simulink model "controller_2022"  (R2022b)
settings: Solver=ode4  StartTime=0.0  StopTime=500  FixedStep=0.001  RelTol=1e-3
model workspace (MAT data in the model file):
  x_0 = 0
values from neighbouring files (symbols this model uses):
  mode = 1    [run_sim.m]
  theta_ref = [0; pi/4; pi]    [run_sim.m]
  v_ref = [0;1;1]    [run_sim.m]
  x0 = zeros(21,1)    [eqn_motion.m]    (also in run_sim.m = zeros(22,1))
undefined symbols (not defined in the file or in its folder): para
libraries: simulink x11, cstblocks x3
settings Model: Creator=kiana  LastModifiedBy=kia241
settings DataIOCC: SaveOutput=off  SignalLogging=off  DSMLogging=off  SaveTime=off  ReturnWorkspaceOutputs=off  StateSaveName=xout_sim  TimeSaveName=tout_sim

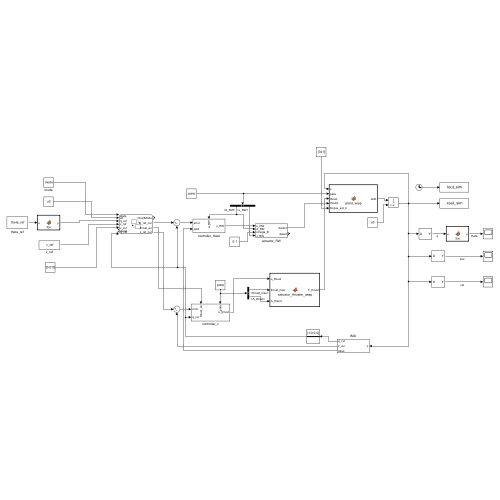
[thumbnail: Simulink's stored preview of the top-level diagram]
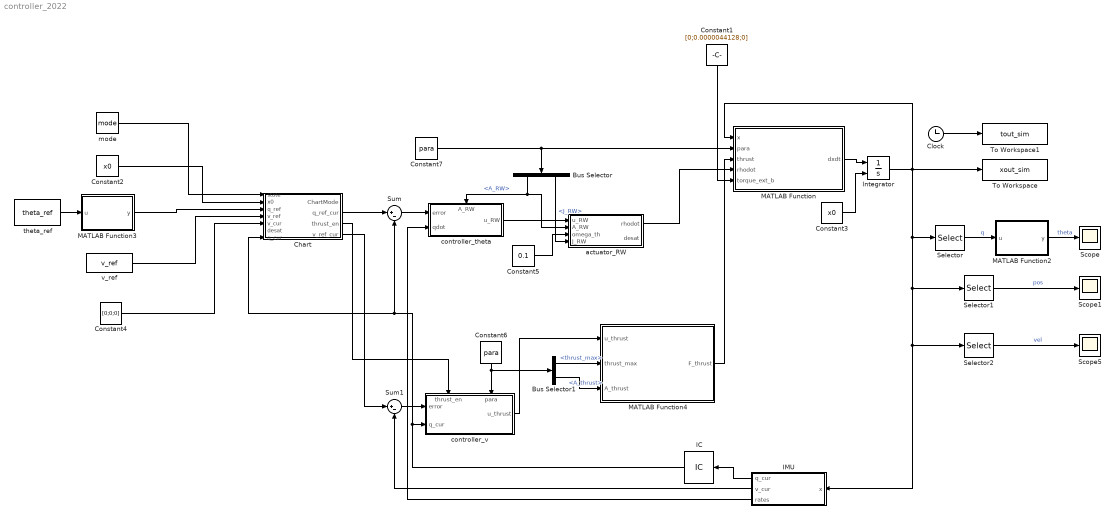
== system controller_2022 ==
  Bus Selector : BusSelector  OutputSignals=A_RW,J_RW
  Bus Selector1 : BusSelector  OutputSignals=thrust_max,A_thrust
  Chart : Stateflow chart  TreatAsAtomicUnit=on
      settings: PortSchema="{\"entries\":[{\"content\":{\"sides\":[{\"content\":{\"connectorIds\":[\"In1\",\"In2\",\"In4\",\"In5\",\"In6\",\"In7\",\"In3\"]},\"type\":\"ConnectorPlacement.EquallySpacedRectSide\",\"uuid\":\"521ec3b6-fc93-445b-ad1f-3cedbe1f933a\"},{\"content\":{\"connectorIds\":[\"Out1\",\"Out2\",\"Out3\",\"Out4\"],\"side\":\"RIGHT\"},\"type\":\"ConnectorPlacement.EquallySpacedRectSide\",\"uuid\":\"d47ee242-db22-486c-9cd8-a97188eab184\"},{\"content\":{\"side\":\"TOP\"},\"type\":\"ConnectorPlacement.EquallySpacedRectSide\",\"uuid\":\"3ac8246c-771a-4a3a-9153-436ad07c67be\"}]},\"type\":\"ConnectorPlacement.EquallySpacedConnector\",\"uuid\":\"e3bfbb62-b6a2-4288-b7fb-0587f308f30e\"}],\"packageUris\":[\"http://schema.mathworks.com/mf0/Connector/R2020b\"],\"version\":\"1.0\"}"
  Clock : Clock
  Constant1 : Constant  Value=[0;0.0000044128;0]
  Constant2 : Constant  Value=x0
  Constant3 : Constant  Value=x0
  Constant4 : Constant  Value=[0;0;0]
  Constant5 : Constant  Value=0.1
  Constant6 : Constant  Value=para  OutDataTypeStr=Bus: para_bus
  Constant7 : Constant  Value=para  OutDataTypeStr=Bus: para_bus
  IC : InitialCondition  Value=[1;0;0;0]
  IMU : Subsystem
  Integrator : Integrator  InitialConditionSource=external  InitialCondition=zeros(21,1)
  MATLAB Function : MATLAB Function  TreatAsAtomicUnit=on
  MATLAB Function2 : MATLAB Function  TreatAsAtomicUnit=on
  MATLAB Function3 : MATLAB Function  TreatAsAtomicUnit=on
  MATLAB Function4 : MATLAB Function  TreatAsAtomicUnit=on
  Scope : Scope
  Scope1 : Scope
  Scope5 : Scope
  Selector : Selector  InputPortWidth=22  IndexOptions=Index vector (dialog)  Indices=[1:4]  OutputSizes=1
  Selector1 : Selector  InputPortWidth=22  IndexOptions=Index vector (dialog)  Indices=[17:19]  OutputSizes=1
  Selector2 : Selector  InputPortWidth=22  IndexOptions=Index vector (dialog)  Indices=[20:22]  OutputSizes=1
  Sum : Sum  Inputs=|+-
  Sum1 : Sum  Inputs=|+-
  To Workspace : ToWorkspace  VariableName=xout_sim  SampleTime=-1
  To Workspace1 : ToWorkspace  VariableName=tout_sim  SampleTime=-1
  actuator_RW : Subsystem
  controller_theta : Subsystem
      settings: PortSchema="{\"entries\":[{\"content\":{\"sides\":[{\"content\":{\"connectorIds\":[\"In1\",\"In2\"]},\"type\":\"ConnectorPlacement.EquallySpacedRectSide\",\"uuid\":\"7526e81d-1261-4d66-9121-bc7373b2004f\"},{\"content\":{\"connectorIds\":[\"Out1\"],\"side\":\"RIGHT\"},\"type\":\"ConnectorPlacement.EquallySpacedRectSide\",\"uuid\":\"2fc2379f-a896-405a-8657-318c2691f466\"},{\"content\":{\"connectorIds\":[\"In3\"],\"side\":\"TOP\"},\"type\":\"ConnectorPlacement.EquallySpacedRectSide\",\"uuid\":\"3ebc5bb4-0a7b-439d-8491-5514c80b6d4e\"}]},\"type\":\"ConnectorPlacement.EquallySpacedConnector\",\"uuid\":\"e4bfc279-4423-461e-be0b-04258d5d0e38\"}],\"packageUris\":[\"http://schema.mathworks.com/mf0/Connector/R2020b\"],\"version\":\"1.0\"}"
  controller_v : Subsystem
      settings: PortSchema="{\"entries\":[{\"content\":{\"sides\":[{\"content\":{\"connectorIds\":[\"In1\",\"In2\"]},\"type\":\"ConnectorPlacement.EquallySpacedRectSide\",\"uuid\":\"7526e81d-1261-4d66-9121-bc7373b2004f\"},{\"content\":{\"connectorIds\":[\"Out1\"],\"side\":\"RIGHT\"},\"type\":\"ConnectorPlacement.EquallySpacedRectSide\",\"uuid\":\"2fc2379f-a896-405a-8657-318c2691f466\"},{\"content\":{\"connectorIds\":[\"In3\",\"In4\"],\"side\":\"TOP\"},\"type\":\"ConnectorPlacement.EquallySpacedRectSide\",\"uuid\":\"3ebc5bb4-0a7b-439d-8491-5514c80b6d4e\"}]},\"type\":\"ConnectorPlacement.EquallySpacedConnector\",\"uuid\":\"e4bfc279-4423-461e-be0b-04258d5d0e38\"}],\"packageUris\":[\"http://schema.mathworks.com/mf0/Connector/R2020b\"],\"version\":\"1.0\"}"
  mode : Constant  Value=mode
  theta_ref : Constant  Value=theta_ref
  v_ref : Constant  Value=v_ref
  wires:
  MATLAB Function/1(dxdt) -> Integrator/1
  MATLAB Function2/1(y) -> Scope/1  "theta"
  Constant3/1 -> Integrator/2
  Selector1/1 -> Scope1/1  "pos"
  Integrator/1 -> Selector2/1, IMU/1(x), Selector1/1, Selector/1, MATLAB Function/1(x), To Workspace/1
  IC/1 -> Chart/3(q_cur), Sum/2, controller_v/2(q_cur)
  Sum/1 -> controller_theta/1(error)
  controller_theta/1(u_RW) -> actuator_RW/1(u_RW)
  IMU/3(rates) -> controller_theta/2(qdot)
  v_ref/1 -> Chart/5(v_ref)
  IMU/2(v_cur) -> Sum1/2
  actuator_RW/1(rhodot) -> MATLAB Function/4(rhodot)
  Sum1/1 -> controller_v/1(error)
  Chart/4(v_ref_cur) -> Sum1/1
  mode/1 -> Chart/1(state)
  Constant2/1 -> Chart/2(x0)
  Selector/1 -> MATLAB Function2/1(u)  "q"
  Chart/2(q_ref_cur) -> Sum/1
  theta_ref/1 -> MATLAB Function3/1(u)
  MATLAB Function3/1(y) -> Chart/4(q_ref)
  IMU/1(q_cur) -> IC/1
  Constant1/1 -> MATLAB Function/5(torque_ext_b)
  Clock/1 -> To Workspace1/1
  MATLAB Function4/1(F_thrust) -> MATLAB Function/3(thrust)
  Selector2/1 -> Scope5/1  "vel"
  controller_v/1(u_thrust) -> MATLAB Function4/1(u_thrust)
  Chart/3(thrust_en) -> controller_v/3(thrust_en)
  Constant4/1 -> Chart/6(v_cur)
  Constant5/1 -> actuator_RW/3(omega_th)
  Constant7/1 -> MATLAB Function/2(para), Bus Selector/1
  Constant6/1 -> Bus Selector1/1, controller_v/4(para)
  Bus Selector/1 -> actuator_RW/2(A_RW), controller_theta/3(A_RW)  "<A_RW>"
  Bus Selector1/1 -> MATLAB Function4/2(thrust_max)  "<thrust_max>"
  Bus Selector1/2 -> MATLAB Function4/3(A_thrust)  "<A_thrust>"
  Bus Selector/2 -> actuator_RW/4(J_RW)  "<J_RW>"

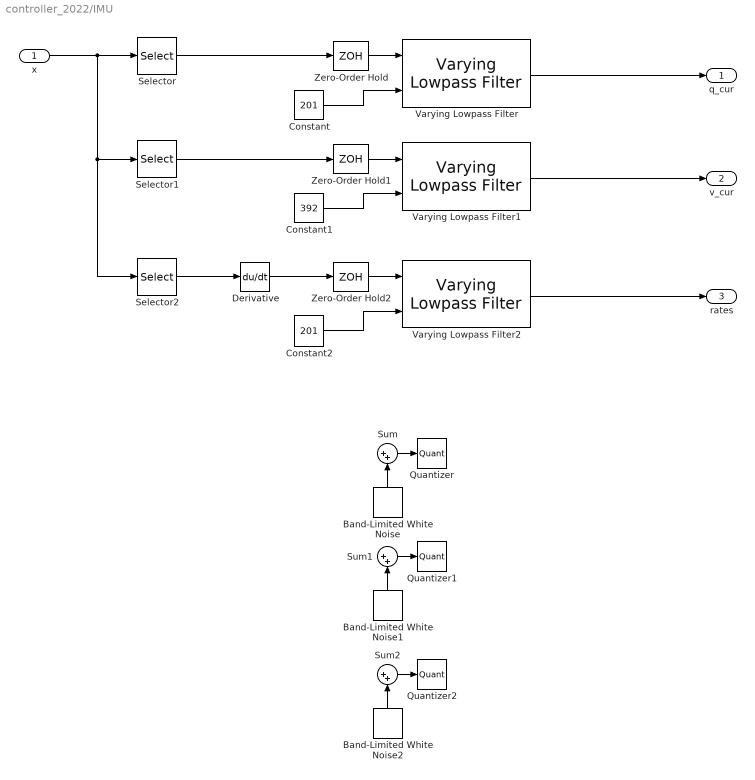
== system controller_2022/IMU ==
  x : Inport
  Band-Limited White Noise : simulink/Sources/Band-Limited White Noise  Cov=[0.1]  Ts=0.1  seed=[23341]
  Band-Limited White Noise1 : simulink/Sources/Band-Limited White Noise  Cov=[0.1]  Ts=0.1  seed=[23341]
  Band-Limited White Noise2 : simulink/Sources/Band-Limited White Noise  Cov=[0.1]  Ts=0.1  seed=[23341]
  Constant : Constant  Value=201
  Constant1 : Constant  Value=392
  Constant2 : Constant  Value=201
  Derivative : Derivative
  Quantizer : Quantizer
  Quantizer1 : Quantizer
  Quantizer2 : Quantizer
  Selector : Selector  InputPortWidth=22  IndexOptions=Index vector (dialog)  Indices=[1:4]  OutputSizes=1
  Selector1 : Selector  InputPortWidth=22  IndexOptions=Index vector (dialog)  Indices=[20:22]  OutputSizes=1
  Selector2 : Selector  InputPortWidth=22  IndexOptions=Index vector (dialog)  Indices=[1:4]  OutputSizes=1
  Sum : Sum  Inputs=|++
  Sum1 : Sum  Inputs=|++
  Sum2 : Sum  Inputs=|++
  Varying Lowpass Filter : cstblocks/Linear Parameter Varying/Varying Lowpass Filter  N=1
  Varying Lowpass Filter1 : cstblocks/Linear Parameter Varying/Varying Lowpass Filter  N=1
  Varying Lowpass Filter2 : cstblocks/Linear Parameter Varying/Varying Lowpass Filter  N=1
  Zero-Order Hold : ZeroOrderHold  SampleTime=0.01
  Zero-Order Hold1 : ZeroOrderHold  SampleTime=0.01
  Zero-Order Hold2 : ZeroOrderHold  SampleTime=0.01
  q_cur : Outport
  v_cur : Outport  Port=2
  rates : Outport  Port=3
  wires:
  x/1 -> Selector2/1, Selector1/1, Selector/1
  Selector/1 -> Zero-Order Hold/1
  Zero-Order Hold/1 -> Varying Lowpass Filter/1
  Constant/1 -> Varying Lowpass Filter/2
  Selector1/1 -> Zero-Order Hold1/1
  Zero-Order Hold1/1 -> Varying Lowpass Filter1/1
  Constant1/1 -> Varying Lowpass Filter1/2
  Constant2/1 -> Varying Lowpass Filter2/2
  Zero-Order Hold2/1 -> Varying Lowpass Filter2/1
  Selector2/1 -> Derivative/1
  Derivative/1 -> Zero-Order Hold2/1
  Sum/1 -> Quantizer/1
  Band-Limited White Noise/1 -> Sum/2
  Sum1/1 -> Quantizer1/1
  Band-Limited White Noise1/1 -> Sum1/2
  Sum2/1 -> Quantizer2/1
  Band-Limited White Noise2/1 -> Sum2/2
  Varying Lowpass Filter/1 -> q_cur/1
  Varying Lowpass Filter1/1 -> v_cur/1
  Varying Lowpass Filter2/1 -> rates/1

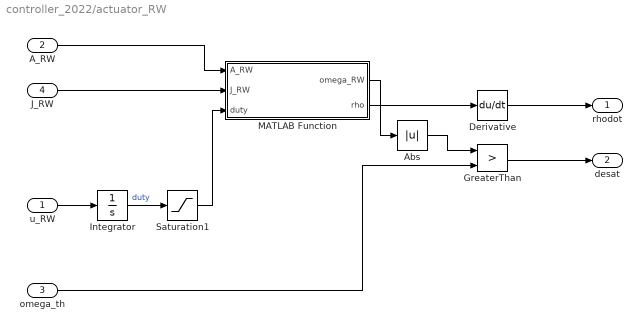
== system controller_2022/actuator_RW ==
  u_RW : Inport
  A_RW : Inport  Port=2
  omega_th : Inport  Port=3
  J_RW : Inport  Port=4
  Abs : Abs  SaturateOnIntegerOverflow=off
  Derivative : Derivative
  GreaterThan : RelationalOperator  Operator=>  OutDataTypeStr=boolean  RndMeth=Simplest  InputSameDT=off
  Integrator : Integrator  InitialCondition=0.15
  MATLAB Function : MATLAB Function  TreatAsAtomicUnit=on
  Saturation1 : Saturate  UpperLimit=0.2  LowerLimit=0.1
  rhodot : Outport
  desat : Outport  Port=2
  wires:
  omega_th/1 -> GreaterThan/2
  GreaterThan/1 -> desat/1
  A_RW/1 -> MATLAB Function/1(A_RW)
  MATLAB Function/2(rho) -> Derivative/1
  Derivative/1 -> rhodot/1
  J_RW/1 -> MATLAB Function/2(J_RW)
  MATLAB Function/1(omega_RW) -> Abs/1
  Abs/1 -> GreaterThan/1
  Integrator/1 -> Saturation1/1  "duty"
  Saturation1/1 -> MATLAB Function/3(duty)
  u_RW/1 -> Integrator/1

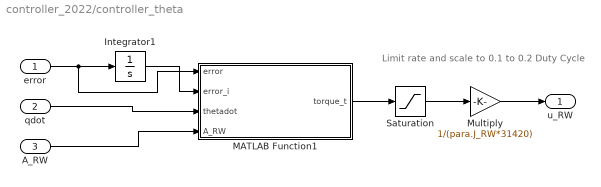
== system controller_2022/controller_theta ==
  note: Limit rate and scale to 0.1 to 0.2 Duty Cycle
  error : Inport
  qdot : Inport  Port=2
  A_RW : Inport  Port=3
  Integrator1 : Integrator  InitialCondition=[0;0;0;0]
  MATLAB Function1 : MATLAB Function  TreatAsAtomicUnit=on
  Multiply : Gain  Gain=1/(para.J_RW*31420)
  Saturation : Saturate  UpperLimit=0.018  LowerLimit=-0.018
  u_RW : Outport
  wires:
  error/1 -> Integrator1/1, MATLAB Function1/1(error)
  Integrator1/1 -> MATLAB Function1/2(error_i)
  A_RW/1 -> MATLAB Function1/4(A_RW)
  qdot/1 -> MATLAB Function1/3(thetadot)
  MATLAB Function1/1(torque_t) -> Saturation/1
  Multiply/1 -> u_RW/1
  Saturation/1 -> Multiply/1

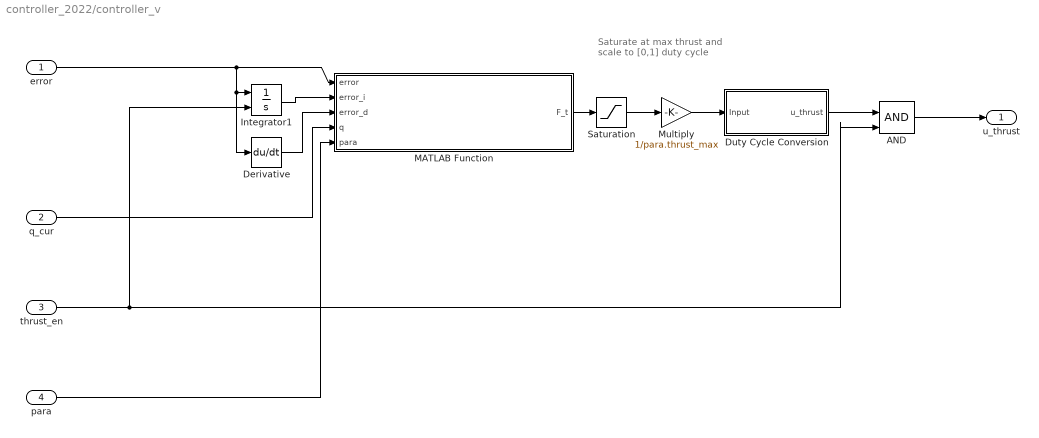
== system controller_2022/controller_v ==
  note: Saturate at max thrust and scale to [0,1] duty cycle
  error : Inport
  q_cur : Inport  Port=2
  thrust_en : Inport  Port=3
  para : Inport  Port=4
  AND : Logic  IconShape=distinctive  AllPortsSameDT=off  OutDataTypeStr=boolean
  Derivative : Derivative
  Duty Cycle Conversion : Subsystem
  Integrator1 : Integrator  ExternalReset=rising  InitialCondition=[0;0;0]
  MATLAB Function : MATLAB Function  TreatAsAtomicUnit=on
  Multiply : Gain  Gain=1/para.thrust_max
  Saturation : Saturate  UpperLimit=para.thrust_max  LowerLimit=0
  u_thrust : Outport
  wires:
  error/1 -> Derivative/1, Integrator1/1, MATLAB Function/1(error)
  Integrator1/1 -> MATLAB Function/2(error_i)
  Derivative/1 -> MATLAB Function/3(error_d)
  q_cur/1 -> MATLAB Function/4(q)
  MATLAB Function/1(F_t) -> Saturation/1
  AND/1 -> u_thrust/1
  Duty Cycle Conversion/1(u_thrust) -> AND/1
  thrust_en/1 -> Integrator1/2, AND/2
  Saturation/1 -> Multiply/1
  Multiply/1 -> Duty Cycle Conversion/1(Input)
  para/1 -> MATLAB Function/5(para)

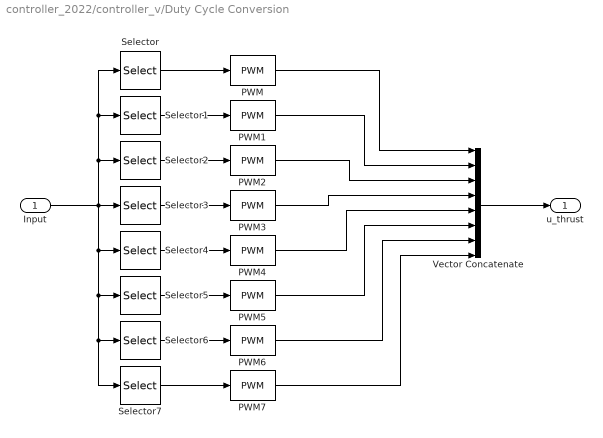
== system controller_2022/controller_v/Duty Cycle Conversion ==
  Input : Inport
  PWM : simulink/Discontinuities/PWM  DisableCoverage=on  Period=0.2  InitialDelay=0  DisallowZeroDutyCycle=off  RunAtFixedTimeIntervals=on  SampleTime=0.001
  PWM{1..7} (7 alike) : simulink/Discontinuities/PWM  DisableCoverage=on  Period=0.2  InitialDelay=0  DisallowZeroDutyCycle=off  RunAtFixedTimeIntervals=on  SampleTime=0.002
  Selector : Selector  InputPortWidth=8  IndexOptions=Index vector (dialog)  Indices=1  OutputSizes=1
  Selector1 : Selector  InputPortWidth=8  IndexOptions=Index vector (dialog)  Indices=2  OutputSizes=1
  Selector2 : Selector  InputPortWidth=8  IndexOptions=Index vector (dialog)  Indices=3  OutputSizes=1
  Selector3 : Selector  InputPortWidth=8  IndexOptions=Index vector (dialog)  Indices=4  OutputSizes=1
  Selector4 : Selector  InputPortWidth=8  IndexOptions=Index vector (dialog)  Indices=5  OutputSizes=1
  Selector5 : Selector  InputPortWidth=8  IndexOptions=Index vector (dialog)  Indices=6  OutputSizes=1
  Selector6 : Selector  InputPortWidth=8  IndexOptions=Index vector (dialog)  Indices=7  OutputSizes=1
  Selector7 : Selector  InputPortWidth=8  IndexOptions=Index vector (dialog)  Indices=8  OutputSizes=1
  Vector Concatenate : Concatenate  NumInputs=8
  u_thrust : Outport
  wires:
  Vector Concatenate/1 -> u_thrust/1
  PWM3/1 -> Vector Concatenate/4
  PWM4/1 -> Vector Concatenate/5
  Selector/1 -> PWM/1
  Selector6/1 -> PWM6/1
  Selector3/1 -> PWM3/1
  PWM6/1 -> Vector Concatenate/7
  Selector5/1 -> PWM5/1
  Selector4/1 -> PWM4/1
  PWM/1 -> Vector Concatenate/1
  Selector2/1 -> PWM2/1
  PWM5/1 -> Vector Concatenate/6
  Selector7/1 -> PWM7/1
  Selector1/1 -> PWM1/1
  PWM7/1 -> Vector Concatenate/8
  PWM2/1 -> Vector Concatenate/3
  Input/1 -> Selector1/1, Selector/1, Selector2/1, Selector7/1, Selector6/1, Selector5/1, Selector4/1, Selector3/1
  PWM1/1 -> Vector Concatenate/2

== stateflow chart controller_2022/Chart ==
  state Reset
    q_ref_cur = x0(1:4);
    v_ref_cur = x0(20:22);
    thrust_en = 0;
  state Drift
    thrust_en = 0;
    q_t = maneuver_slew_wrap(v_cur, v_ref);
  state Desat
    thrust_en = 1;
    v_ref_cur = 0;
  state Slew
    q_ref_cur=q_ref;
    thrust_en = 0;
  state Maneuver_slew
    q_ref_cur = q_t;
    thrust_en = 0;
  state Maneuver_v
    q_ref_cur = q_t;
    v_ref_cur=v_ref;
    thrust_en = 1;
  (default) -> Reset
  Reset -> Drift
  Drift -> Desat [order 3] : [desat==1]
  Drift -> Slew [order 2] : [state == 1]
  Drift -> Maneuver_slew [order 1] : [state == 2]
  Maneuver_slew -> Maneuver_v : [abs(q_cur - q_ref_cur)<0.01]
  data: v_cur_in function_input; v_ref_in function_input; out function_output; ChartMode output Enum: ChartModeType; state input size=1; x0 input; q_cur input size=4; q_ref input size=4; q_t local size=4; q_ref_cur output size=4; v_ref input; thrust_en output; v_ref_cur output; v_cur input; desat input
  function out = maneuver_slew_wrap(v_cur_in, v_ref_in):
    | function out = maneuver_slew_wrap(v_cur_in, v_ref_in)
    |     out = maneuver_slew(v_cur_in, v_ref_in);
    | end

== matlab function controller_2022/controller_v/MATLAB Function ==
  data: error input; F_t output; error_i input; error_d input; q input; para input
function F_t = control_v_PID_wrap(error, error_i, error_d, q, para)
    F_t = control_x_PID(error, error_i, error_d, q, para);
end

== matlab function controller_2022/MATLAB Function2 ==
  data: u input; y output
function y = fcn(u)
    y = transpose(flip(quat2eul(u'))); %returns [phi; theta; psi]
end

== matlab function controller_2022/MATLAB Function3 ==
  data: u input; y output
function y = fcn(u)
    y = eul2quat(flip(u)');
end

== matlab function controller_2022/MATLAB Function4 ==
  data: u_thrust input; F_thrust output; thrust_max input; A_thrust input
function F_thrust = actuator_thruster_wrap(u_thrust, thrust_max, A_thrust)
    F_thrust = actuator_thruster(u_thrust, thrust_max, A_thrust);
end

== matlab function controller_2022/actuator_RW/MATLAB Function ==
  data: A_RW input; J_RW input; duty input; omega_RW output; rho output
function [omega_RW, rho] = actuator_RW_wrap(A_RW, J_RW,duty)
    [omega_RW, rho] = actuator_RW(A_RW, J_RW, duty);
end

== matlab function controller_2022/MATLAB Function ==
  settings: updateMethod=DISCRETE  sampleTime=0.001
  data: x input size=22; para input; dxdt output size=22; thrust input; rhodot input; torque_ext_b input
function dxdt= plant_wrap(x, para, thrust, rhodot, torque_ext_b)
    coder.extrinsic('Simulink.Bus');
    %para.m = m;
    %para.x_cm = x_cm;
    %para.x_nozzle = x_nozzle;
    %para.I = I;
    dxdt = plant(x, para, thrust, rhodot, torque_ext_b);
end

== matlab function controller_2022/controller_theta/MATLAB Function1 ==
  data: error input; torque_t output; error_i input; thetadot input; A_RW input
function torque_t = theta_PID_wrap(error, error_i, thetadot, A_RW)
    torque_t = control_theta_PID(error, error_i, thetadot, A_RW);
end
